simulink model "collision"  (Simulink 9.2)
settings: Solver=VariableStepAuto  StartTime=0.0  StopTime=50  RelTol=1e-3
settings Model: Creator=jinwooro  LastModifiedBy=jinwooro
settings DataIOCC: LimitDataPoints=off  SaveFormat=Dataset  SignalLoggingSaveFormat=Dataset
settings OptimizationCC: LifeSpan=auto
settings DebuggingCC: UnderspecifiedInitializationDetection=Simplified  MergeDetectMultiDrivingBlocksExec=error  FcnCallInpInsideContextMsg=error  StateNameClashWarn=none  SFUnexpectedBacktrackingDiag=error  SFNoUnconditionalDefaultTransitionDiag=error  SFExecutionAtInitializationDiag=warning
settings HardwareCC: ProdBitPerPointer=64  ProdBitPerSizeT=64  ProdBitPerPtrDiffT=64  ProdLargestAtomicFloat=Float  ProdIntDivRoundTo=Zero  ProdEndianess=LittleEndian  ProdWordSize=64  ProdHWDeviceType=Intel->x86-64 (Windows64)
settings ModelReferenceCC: PropagateSignalLabelsOutOfModel=on
settings SFSimCC: SimUseLocalCustomCode=on
settings RTWCC: RTWUseLocalCustomCode=on
settings CodeAppCC: StateflowObjectComments=off
settings GRTTargetCC: TargetLangStandard=C99 (ISO)  GeneratePreprocessorConditionals=Use local settings  CombineOutputUpdateFcns=on  GRTInterface=off
settings ConfigComp: CovMetricSettings=dwe  CovHtmlReporting=off  CovSaveCumulativeToWorkspaceVar=off  CovSaveSingleToWorkspaceVar=off  CovExternalEMLEnable=on

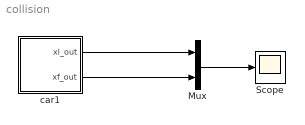
== system collision ==
  Mux : Mux  Inputs=2
  Scope : Scope
  car1 : Stateflow chart  TreatAsAtomicUnit=on
  wires:
  Mux/1 -> Scope/1
  car1/1(xl_out) -> Mux/1
  car1/2(xf_out) -> Mux/2

== stateflow chart car1 ==
  settings: updateMethod=CONTINUOUS
  state Driving
    du:
    T_dot = 1;
    xl_dot = 7 * sin(0.5 * T) + 7;
    xf_dot = 0.9 * (xl - xf);
    xl_out = xl;
    xf_out = xf;
  state Violation
    du:
    T_dot = 1;
    xl_dot = 7 * sin(0.5 * T) + 7;
    xf_dot = 0;
    xf_out = xf;
    xl_out = xl;
  (default) -> Driving : {
      | xl = 30;
      | xf = 0;
      | T = 0;
      | }
  Driving -> Violation : [power(xl - xf - 2, 0.5) <= 2]
  Violation -> Driving : [power(xl - xf - 5, 0.5) >= 2]
  data: xf local double; xl_out output double; T local double; xl local double; xf_out output double
  data xf settings: updateMethod=SF_CONTINUOUS_TIME_DATA
  data T settings: updateMethod=SF_CONTINUOUS_TIME_DATA
  data xl settings: updateMethod=SF_CONTINUOUS_TIME_DATA
